simulink model "SystemSimulinkModel"  (R2024b)
settings: Solver=VariableStepAuto  StartTime=0.0  StopTime=10.0  RelTol=1e-3
values from neighbouring files (symbols this model uses):
  Km = 182.7    [MotorCharacterization.m]
  Kp = 1000    [MotorCharacterization.m]
  tau = 50*10^(-3)    (= 0.05)    [MotorCharacterization.m]
  V = 5    [MotorCharacterization.m]
settings Model: Creator=fsant  LastModifiedBy=fsant

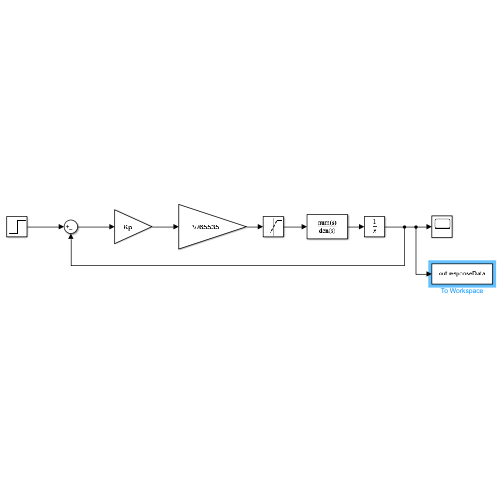
[thumbnail: Simulink's stored preview of the top-level diagram]
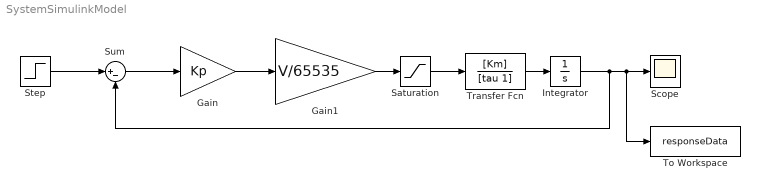
== system SystemSimulinkModel ==
  Gain : Gain  Gain=Kp
  Gain1 : Gain  Gain=V/65535
  Integrator : Integrator
  Saturation : Saturate  UpperLimit=V  LowerLimit=-V
  Scope : Scope
  Step : Step  Time=0  After=500  SampleTime=0.001
  Sum : Sum  Inputs=|+-
  To Workspace : ToWorkspace  VariableName=responseData  SampleTime=-1
  Transfer Fcn : TransferFcn  Numerator=[Km]  Denominator=[tau 1]
  wires:
  Gain/1 -> Gain1/1
  Gain1/1 -> Saturation/1
  Sum/1 -> Gain/1
  Saturation/1 -> Transfer Fcn/1
  Transfer Fcn/1 -> Integrator/1
  Integrator/1 -> Sum/2, To Workspace/1, Scope/1
  Step/1 -> Sum/1
